simulink model "testing_DM_hby"  (R2023b)
settings: Solver=FixedStepDiscrete  StartTime=0.0  StopTime=inf  FixedStep=0.003  RelTol=1e-3
InitFcn:
  | run('/home/uonaim/matlab_ws/FOOT/joint_calibration.m');
undefined symbols (not defined in the file or in its folder): CAL
libraries: ros2lib x12
(part 2 of 2)

== matlab function testing_DM_hby/Foot_Home_Then_Sine ==
  data: t input; x_cmd output; sequence_enable input; x_actual input; y_actual input; x_home input; y_home input; home_duration input; home_tolerance input; settle_time input; path_width input; amplitude input; period input; y_cmd output; phase output; home_reached output; trajectory_active output; valid output
function [x_cmd, y_cmd, phase, home_reached, ...
          trajectory_active, valid] = ...
    Foot_Home_Then_Sine( ...
    t, sequence_enable, x_actual, y_actual, ...
    x_home, y_home, home_duration, ...
    home_tolerance, settle_time, ...
    path_width, amplitude, period)
%#codegen
%
% right switch启动后：
% phase=0：未启动，目标跟随实际位置
% phase=1：平滑移动到预定起点
% phase=2：从预定起点开始正弦往返轨迹
%
% 坐标单位：m
% 时间单位：s

persistent state
persistent last_enable
persistent t_phase_start
persistent x_begin
persistent y_begin
persistent tolerance_start_time

if isempty(state)
    state = uint8(0);
    last_enable = false;

    t_phase_start = 0.0;
    x_begin = single(0.0);
    y_begin = single(0.0);

    tolerance_start_time = -1.0;
end

%% 类型转换

t = double(t);

enable = sequence_enable ~= 0;

x_actual = single(x_actual);
y_actual = single(y_actual);

x_home = single(x_home);
y_home = single(y_home);

home_duration  = single(home_duration);
home_tolerance = single(home_tolerance);
settle_time    = single(settle_time);

path_width = single(path_width);
amplitude  = single(amplitude);
period     = single(period);

%% 默认输出

x_cmd = x_actual;
y_cmd = y_actual;

phase = state;

home_reached = false;
trajectory_active = false;
valid = false;

%% 输入有效性检查

input_valid = ...
    isfinite(x_actual) && ...
    isfinite(y_actual) && ...
    isfinite(x_home) && ...
    isfinite(y_home) && ...
    isfinite(home_duration) && ...
    isfinite(home_tolerance) && ...
    isfinite(settle_time) && ...
    isfinite(path_width) && ...
    isfinite(amplitude) && ...
    isfinite(period);

if ~input_valid
    state = uint8(0);
    last_enable = false;
    return;
end

if home_duration <= single(0.01) || ...
   home_tolerance <= single(0.0) || ...
   settle_time < single(0.0) || ...
   period <= single(0.01)

    state = uint8(0);
    last_enable = false;
    return;
end

valid = true;

%% sequence关闭：目标保持在当前实际位置，并复位状态机

if ~enable
    state = uint8(0);
    last_enable = false;

    tolerance_start_time = -1.0;

    x_cmd = x_actual;
    y_cmd = y_actual;

    phase = uint8(0);
    return;
end

%% 检测right switch启动上升沿

if enable && ~last_enable
    state = uint8(1);

    t_phase_start = t;

    % 记录启动瞬间的真实位置
    x_begin = x_actual;
    y_begin = y_actual;

    tolerance_start_time = -1.0;
end

last_enable = true;

%% 状态1：平滑回到指定起点

if state == uint8(1)

    elapsed = t - t_phase_start;

    u = elapsed / double(home_duration);

    if u < 0.0
        u = 0.0;
    elseif u > 1.0
        u = 1.0;
    end

    % 半余弦平滑插值：
    % 起点、终点速度均为0
    blend = 0.5 - 0.5*cos(pi*u);

    x_cmd = x_begin + ...
        (x_home - x_begin)*single(blend);

    y_cmd = y_begin + ...
        (y_home - y_begin)*single(blend);

    phase = uint8(1);

    % 插值结束后，等待实际位置真正到达
    if u >= 1.0

        position_error = sqrt( ...
            (x_actual-x_home)*(x_actual-x_home) + ...
            (y_actual-y_home)*(y_actual-y_home));

        if position_error <= home_tolerance

            if tolerance_start_time < 0.0
                tolerance_start_time = t;
            end

            % 必须连续稳定一段时间才进入正弦阶段
            if (t-tolerance_start_time) >= double(settle_time)

                state = uint8(2);
                t_phase_start = t;

                x_cmd = x_home;
                y_cmd = y_home;

                phase = uint8(2);
                home_reached = true;
            end
        else
            tolerance_start_time = -1.0;
        end
    end

    return;
end

%% 状态2：绘制正弦往返轨迹

if state == uint8(2)

    home_reached = true;
    trajectory_active = true;
    phase = uint8(2);

    tau = t - t_phase_start;

    if tau < 0.0
        tau = 0.0;
    end

    tau_cycle = mod(tau, double(period));

    % s：0 → 1 → 0
    s = 0.5 - ...
        0.5*cos(2.0*pi*tau_cycle/double(period));

    s_single = single(s);

    x_cmd = x_home + path_width*s_single;

    y_cmd = y_home + ...
        amplitude*sin(single(2.0*pi)*s_single);

    return;
end

%% 异常状态保护

state = uint8(0);
phase = uint8(0);

x_cmd = x_actual;
y_cmd = y_actual;

valid = false;

end

== matlab function testing_DM_hby/FiveBar_IK ==
  data: x_cmd input; alpha_cmd output; y_cmd input; L1 input; L2 input; L3 input; L4 input; L5 input; alpha_ref input; beta_ref input; beta_cmd output; valid output
function [alpha_cmd, beta_cmd, valid] = fivebar_ik( ...
    x_cmd, y_cmd, L1, L2, L3, L4, L5, ...
    alpha_ref, beta_ref)
%#codegen
%
% 平面五连杆逆运动学
%
% 坐标系：
% 左侧固定关节 O = (0,0)
% 右侧固定关节 D = (L5,0)
% x 向右为正
% y 向下为正
%
% 长度单位：m
% 角度单位：rad

alpha_cmd = alpha_ref;
beta_cmd  = beta_ref;
valid = false;

eps_r = single(1.0e-6);

%% 左侧两连杆

rx1 = x_cmd;
ry1 = y_cmd;

r1 = sqrt(rx1 * rx1 + ry1 * ry1);

if r1 < eps_r
    return;
end

c_alpha = ...
    (r1 * r1 + L1 * L1 - L2 * L2) / ...
    (single(2.0) * L1 * r1);

if c_alpha > single(1.0) || c_alpha < single(-1.0)
    return;
end

c_alpha = min(max(c_alpha, single(-1.0)), single(1.0));

phi1 = atan2(ry1, rx1);
delta1 = acos(c_alpha);

alpha_1 = phi1 + delta1;
alpha_2 = phi1 - delta1;

err_alpha_1 = abs(atan2( ...
    sin(alpha_1 - alpha_ref), ...
    cos(alpha_1 - alpha_ref)));

err_alpha_2 = abs(atan2( ...
    sin(alpha_2 - alpha_ref), ...
    cos(alpha_2 - alpha_ref)));

if err_alpha_1 <= err_alpha_2
    alpha_cmd = alpha_1;
else
    alpha_cmd = alpha_2;
end

%% 右侧两连杆

rx2 = x_cmd - L5;
ry2 = y_cmd;

r2 = sqrt(rx2 * rx2 + ry2 * ry2);

if r2 < eps_r
    return;
end

c_beta = ...
    (r2 * r2 + L4 * L4 - L3 * L3) / ...
    (single(2.0) * L4 * r2);

if c_beta > single(1.0) || c_beta < single(-1.0)
    return;
end

c_beta = min(max(c_beta, single(-1.0)), single(1.0));

phi2 = atan2(ry2, rx2);
delta2 = acos(c_beta);

beta_1 = phi2 + delta2;
beta_2 = phi2 - delta2;

err_beta_1 = abs(atan2( ...
    sin(beta_1 - beta_ref), ...
    cos(beta_1 - beta_ref)));

err_beta_2 = abs(atan2( ...
    sin(beta_2 - beta_ref), ...
    cos(beta_2 - beta_ref)));

if err_beta_1 <= err_beta_2
    beta_cmd = beta_1;
else
    beta_cmd = beta_2;
end

valid = true;

end

== matlab function testing_DM_hby/FiveBar_Animation ==
  data: time_in input; alpha input; beta input; xB input; yB input; L1 input; L4 input; L5 input; valid input
function FiveBar_Animation( ...
    time_in, alpha, beta, xB, yB, L1, L4, L5, valid)
%#codegen

coder.extrinsic('fivebar_plot_smooth');

if coder.target('Sfun')

    fivebar_plot_smooth( ...
        double(time_in), ...
        double(alpha), ...
        double(beta), ...
        double(xB), ...
        double(yB), ...
        double(L1), ...
        double(L4), ...
        double(L5), ...
        logical(valid));

end

end

== matlab function testing_DM_hby/Foot_Sine_Trajectory ==
  data: time_in input; x_cmd output; enable_in input; x_center_in input; y_center_in input; width_in input; amplitude_in input; period_in input; y_cmd output; s output
function [x_cmd, y_cmd, s] = foot_sine_trajectory( ...
    time_in, enable_in, ...
    x_center_in, y_center_in, ...
    width_in, amplitude_in, period_in)
%#codegen
%
% 足端正弦轨迹发生器
%
% 输出：
% x_cmd、y_cmd：目标足端位置，单位 m
% s：轨迹参数，范围 0～1～0
%
% 坐标系：
% x 向右为正
% y 向下为正

%% 强制内部采用 single

t = single(time_in);

x_center = single(x_center_in);
y_center = single(y_center_in);

width     = single(width_in);
amplitude = single(amplitude_in);
period    = single(period_in);

pi_s = single(3.14159265358979323846);
half = single(0.5);
one  = single(1.0);

%% 默认输出中心点

x_cmd = x_center;
y_cmd = y_center;
s = single(0.0);

%% 未启用或周期无效时保持中心点

if ~logical(enable_in)
    return;
end

if period <= single(1.0e-3)
    return;
end

%% 平滑往返轨迹参数

omega = single(2.0) * pi_s / period;

s = half - half * cos(omega * t);

%% 正弦足端轨迹

x_cmd = x_center + width * (s - half);

y_cmd = y_center + amplitude * ...
    sin(single(2.0) * pi_s * s);

end

== matlab function testing_DM_hby/Left_Joint_To_Motor ==
  data: alpha_cmd input; p_LA_target output; beta_cmd input; p_LB_target output; valid output
function [p_LA_target, p_LB_target, valid] = ...
    Left_Joint_To_Motor(alpha_cmd, beta_cmd)
%#codegen
% 左腿关节目标角转换为达妙电机目标角
%
% 标定关系：
% q_joint = (q_motor - qm0) * sign / ratio + qj0
%
% 逆变换：
% q_motor = qm0 + (q_joint - qj0) * ratio / sign

qm0_LA   = single(-0.3408479690551758);
qj0_LA   = single( 3.504545610856599);
sign_LA  = single(-1.0);
ratio_LA = single( 1.0);

qm0_LB   = single(-0.6292438507080078);
qj0_LB   = single( 0.8999130837716534);
sign_LB  = single(-1.0);
ratio_LB = single( 1.0);

alpha_cmd = single(alpha_cmd);
beta_cmd  = single(beta_cmd);

p_LA_target = qm0_LA + ...
    (alpha_cmd - qj0_LA) * ratio_LA / sign_LA;

p_LB_target = qm0_LB + ...
    (beta_cmd - qj0_LB) * ratio_LB / sign_LB;

valid = isfinite(p_LA_target) && isfinite(p_LB_target);

end

== matlab function testing_DM_hby/Motor_To_Joint_LA/Motor_Position_To_Joint ==
  data: q_motor input; q_joint output; q_motor_ref input; q_joint_ref input; motor_sign input; motor_ratio input
function q_joint = motor_position_to_joint( ...
    q_motor, q_motor_ref, q_joint_ref, ...
    motor_sign, motor_ratio)
%#codegen
%
% 电机位置反馈转换为运动学关节角
%
% q_motor      当前电机位置反馈，rad
% q_motor_ref  标定参考姿态下的电机位置，rad
% q_joint_ref  标定参考姿态下的模型关节角，rad
% motor_sign   +1 或 -1
% motor_ratio  电机角变化/关节角变化

qm = single(q_motor);
qm0 = single(q_motor_ref);
qj0 = single(q_joint_ref);
sgn = single(motor_sign);
ratio = single(motor_ratio);

q_joint = qj0;

if abs(ratio) > single(1.0e-6)
    q_joint = qj0 + ...
        sgn * (qm - qm0) / ratio;
end

end
